simulink model "Powertrain_Model"  (R2021b)
settings: Solver=VariableStepAuto  StartTime=1  StopTime=sim_time  FixedStep=1  RelTol=1e-3
values from neighbouring files (symbols this model uses):
  a = (1-WD)*L    (= 1.352)    [Master_Script.m]
  airDen = 1.26    [Master_Script.m]
  b = WD*L    (= 1.248)    [Master_Script.m]
  Cd = 0.27    [Master_Script.m]
  contPowerRating = contPowerRating * numMotors    (= 400000)    [Master_Script.m]
  eff_batt = 0.9    [Master_Script.m]
  eff_trans = 0.95    [Master_Script.m]
  EM_Torque_Map = EM_Torque_Map * numMotors    [Master_Script.m]
  EM_Torque_Max = EM_Torque_Max * numMotors    [Master_Script.m]
  fArea = w103Dim*h101Dim    (= 2.727)    [Master_Script.m]
  followDriveCycle = 0    [Master_Script.m]
  fr = 0.009    [Master_Script.m]
  g = 9.81    [Master_Script.m]
  gearRatio = 8    [Master_Script.m]
  grade = 0    [Master_Script.m]    (also in isSetupSuitable.m = 0.12)
  h = 0.65    [Master_Script.m]
  isRWD = 0    [Master_Script.m]
  Ki = 0    [Master_Script.m]
  Kp = 1    [Master_Script.m]
  L = 2.6    [Master_Script.m]
  mu = 1    [Master_Script.m]
  mVehicle = originalmVehicle    (= 1372.4)    [Master_Script.m]
  netBattCap = capCell * numCellSeries * numParallelStrings    (= 52.224)    [Master_Script.m]
  R = 0.6681    [Master_Script.m]
undefined symbols (not defined in the file or in its folder): alpha, EM_Efficiency, EM_Omega_Map, EM_Omega_Max, t_cyc, v_cyc
libraries: slpidlib x1
settings Model: Creator=adity  LastModifiedBy=Shubham
settings SolverCC: AlgebraicLoopSolver=TrustRegion
settings DebuggingCC: SFMachineParentedDataDiag=warning
settings SFSimCC: CustomCodeUndefinedFunction=UseInterfaceOnly

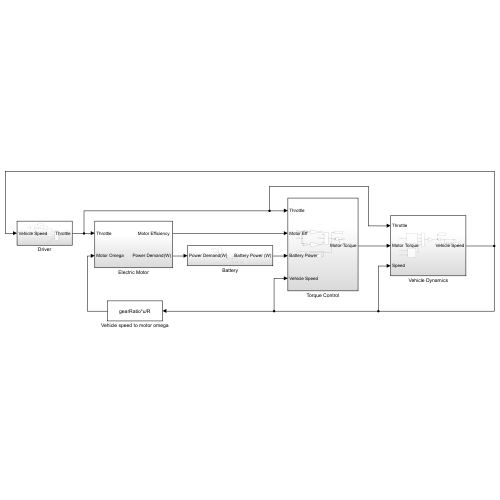
[thumbnail: Simulink's stored preview of the top-level diagram]
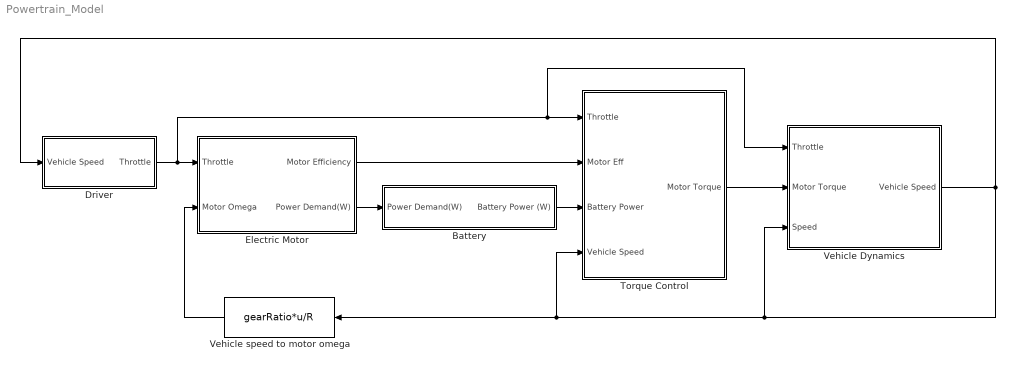
== system Powertrain_Model ==
  Battery : Subsystem
  Driver : Subsystem
  Electric Motor : Subsystem
  Torque Control : Subsystem
  Vehicle Dynamics : Subsystem
  Vehicle speed to motor omega : Fcn  Expr=gearRatio*u/R
  wires:
  Driver/1(Throttle) -> Vehicle Dynamics/1(Throttle), Torque Control/1(Throttle), Electric Motor/1("Throttle ")
  Vehicle speed to motor omega/1 -> Electric Motor/2(Motor Omega)
  Electric Motor/2(Power Demand(W)) -> Battery/1(Power Demand(W))
  Vehicle Dynamics/1(Vehicle Speed) -> Driver/1(Vehicle Speed), Vehicle Dynamics/3(Speed), Torque Control/4(Vehicle Speed), Vehicle speed to motor omega/1
  Battery/1(Battery Power (W)) -> Torque Control/3(Battery Power)
  Electric Motor/1("Motor Efficiency ") -> Torque Control/2(Motor Eff)
  Torque Control/1(Motor Torque) -> Vehicle Dynamics/2(Motor Torque)

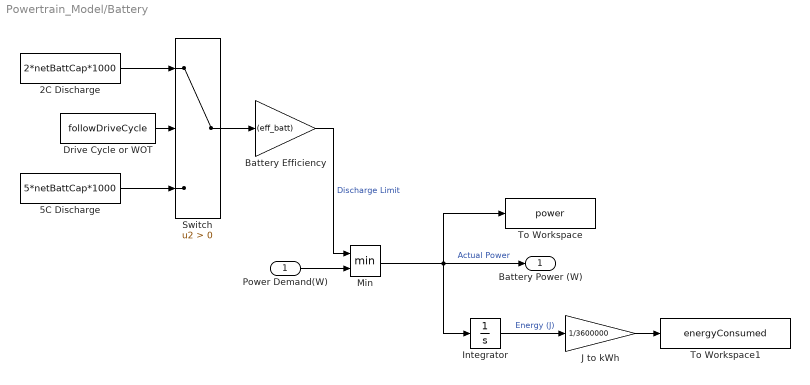
== system Powertrain_Model/Battery ==
  Power Demand(W) : Inport
  2C Discharge : Constant  Value=2*netBattCap*1000
  5C Discharge : Constant  Value=5*netBattCap*1000
  Battery Efficiency : Gain  Gain=(eff_batt)
  Drive Cycle or WOT : Constant  Value=followDriveCycle
  Integrator : Integrator
  J to kWh : Gain  Gain=1/3600000
  Min : MinMax  Inputs=2
  Switch : Switch  Criteria=u2 > Threshold
  To Workspace : ToWorkspace  VariableName=power  SaveFormat=Timeseries  SampleTime=-1
  To Workspace1 : ToWorkspace  VariableName=energyConsumed  SaveFormat=Timeseries  SampleTime=-1
  Battery Power (W) : Outport
  wires:
  Min/1 -> Battery Power (W)/1, To Workspace/1, Integrator/1  "Actual Power"
  Integrator/1 -> J to kWh/1  "Energy (J)"
  J to kWh/1 -> To Workspace1/1
  5C Discharge/1 -> Switch/3
  Battery Efficiency/1 -> Min/1  "Discharge Limit"
  Drive Cycle or WOT/1 -> Switch/2
  Switch/1 -> Battery Efficiency/1
  2C Discharge/1 -> Switch/1
  Power Demand(W)/1 -> Min/2

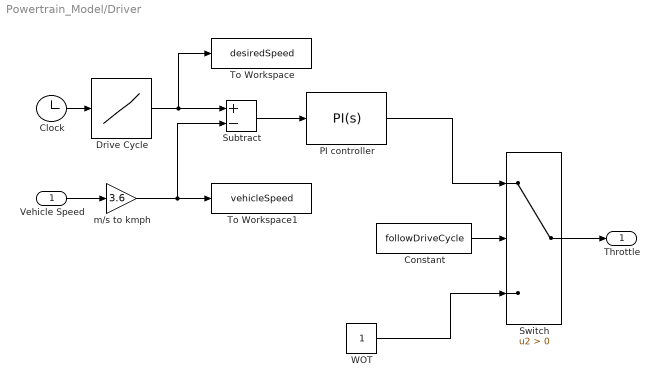
== system Powertrain_Model/Driver ==
  Vehicle Speed : Inport
  Clock : Clock
  Constant : Constant  Value=followDriveCycle
  Drive Cycle : Lookup_n-D  NumberOfTableDimensions=1  BreakpointsForDimension1=t_cyc  Table=v_cyc  InternalRulePriority=Speed  RndMeth=Simplest  InputSameDT=on
  "PI controller " : slpidlib/PID Controller  Controller=PI  Form=Parallel  TimeDomain=Continuous-time  UseExternalTs=off  SampleTime=-1  IntegratorMethod=Forward Euler  FilterMethod=Forward Euler  ControllerParametersSource=internal  P=Kp  I=Ki  D=0  UseFilter=on  N=100  TunerSelectOption=Transfer Function Based (PID Tuner App)  InitialConditionSource=internal  InitialConditionForIntegrator=0  InitialConditionForFilter=0  DifferentiatorICPrevScaledInput=0  ExternalReset=none  TrackingMode=off  Kt=1  LimitOutput=on  SatLimitsSource=internal  UpperSaturationLimit=1  LowerSaturationLimit=-1  LinearizeAsGain=on  AntiWindupMode=none  Kb=1  POutMin=[]  POutMax=[]  IOutMin=[]  IOutMax=[]  DOutMin=[]  DOutMax=[]  NOutMin=[]  NOutMax=[]  SumOutMin=[]  SumOutMax=[]  SaturationOutMin=[]  SaturationOutMax=[]  PParamMin=[]  PParamMax=[]  IParamMin=[]  IParamMax=[]  DParamMin=[]  DParamMax=[]  NParamMin=[]  NParamMax=[]  KbParamMin=[]  KbParamMax=[]  KtParamMin=[]  KtParamMax=[]  KbOutMin=[]  KbOutMax=[]  KtOutMin=[]  KtOutMax=[]  IntegratorOutMin=[]  IntegratorOutMax=[]  FilterOutMin=[]  FilterOutMax=[]  SumI1OutMin=[]  SumI1OutMax=[]  SumI2OutMin=[]  SumI2OutMax=[]  SumI3OutMin=[]  SumI3OutMax=[]  SumI4OutMin=[]  SumI4OutMax=[]  SumDOutMin=[]  SumDOutMax=[]  DifferentiatorOutMin=[]  DifferentiatorOutMax=[]  FilterDiffOutCoefMin=[]  FilterDiffOutCoefMax=[]  ReciprocalOutMin=[]  ReciprocalOutMax=[]  SumDenOutMin=[]  SumDenOutMax=[]  SumNumOutMin=[]  SumNumOutMax=[]  DivideOutMin=[]  DivideOutMax=[]  UdiffTsProdOutMin=[]  UdiffTsProdOutMax=[]  NTsProdOutMin=[]  NTsProdOutMax=[]  UintegralTsProdOutMin=[]  UintegralTsProdOutMax=[]  UngainTsProdOutMin=[]  UngainTsProdOutMax=[]  IntegratorContinuousStateAttributes=''  IntegratorStateMustResolveToSignalObject=off  IntegratorRTWStateStorageClass=Auto  FilterContinuousStateAttributes=''  FilterStateMustResolveToSignalObject=off  FilterRTWStateStorageClass=Auto  ParallelPVariant=InternalParameters  IdealPVariant=Disabled  IVariant=InternalParameters  DVariant=Disabled  IntegratorVariant=Continuous  SatVariant=Enabled  AWVariant=Passthrough  PCopyVariant=Disabled  TRVariant=Disabled  FdbkBlocksVariant=Forward  IdealPFdbkVariant=Disabled  SatFdbkVariant=Disabled  DerivativeFilterVariant=Disabled  NVariant=Disabled  NCopyVariant=Disabled_SignalSpec  FilterICVariant=Disabled  IntegratorICVariant=InternalICs  ExternalResetVariant=Disabled  TRSumVariant=Passthrough  SumFdbkVariant=Disabled  SumVariant=Sum_PI  TsampFilterVariant=InternalTs  TsampNgainVariant=Passthrough  TsampIntegralVariant=Passthrough  ExternalSaturationOutDataTypeStr=Inherit: Same as second input
  Subtract : Sum  Inputs=+-
  Switch : Switch  Criteria=u2 > Threshold
  To Workspace : ToWorkspace  VariableName=desiredSpeed  SaveFormat=Timeseries  SampleTime=-1
      settings: Save2DSignal=2-D array (concatenate along first dimension)
  To Workspace1 : ToWorkspace  VariableName=vehicleSpeed  SaveFormat=Timeseries  SampleTime=-1
  WOT : Constant
  m/s to kmph : Gain  Gain=3.6
  Throttle : Outport
  wires:
  Drive Cycle/1 -> Subtract/1, To Workspace/1
  Subtract/1 -> "PI controller "/1
  Clock/1 -> Drive Cycle/1
  Switch/1 -> Throttle/1
  "PI controller "/1 -> Switch/1
  Constant/1 -> Switch/2
  WOT/1 -> Switch/3
  Vehicle Speed/1 -> m/s to kmph/1
  m/s to kmph/1 -> To Workspace1/1, Subtract/2

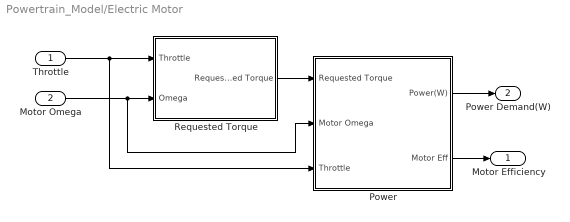
== system Powertrain_Model/Electric Motor ==
  "Throttle " : Inport
  Motor Omega : Inport  Port=2
  Power : Subsystem
  Requested Torque : Subsystem
  "Motor Efficiency " : Outport
  Power Demand(W) : Outport  Port=2
  wires:
  Requested Torque/1(Requested Torque) -> Power/1(Requested Torque)
  "Throttle "/1 -> Requested Torque/1(Throttle), Power/3("Throttle ")
  Power/1("Power(W) ") -> Power Demand(W)/1
  Motor Omega/1 -> Requested Torque/2(Omega), Power/2(Motor Omega)
  Power/2(Motor Eff) -> "Motor Efficiency "/1

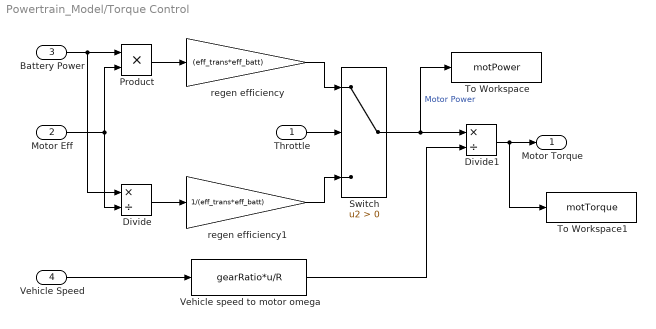
== system Powertrain_Model/Torque Control ==
  Throttle : Inport
  Motor Eff : Inport  Port=2
  Battery Power : Inport  Port=3
  Vehicle Speed : Inport  Port=4
  Divide : Product  Inputs=*/
  Divide1 : Product  Inputs=*/
  Product : Product
  Switch : Switch  Criteria=u2 > Threshold
  To Workspace : ToWorkspace  VariableName=motPower  SaveFormat=Timeseries  SampleTime=-1
  To Workspace1 : ToWorkspace  VariableName=motTorque  SaveFormat=Timeseries  SampleTime=-1
  Vehicle speed to motor omega : Fcn  Expr=gearRatio*u/R
  regen efficiency : Gain  Gain=(eff_trans*eff_batt)
  regen efficiency1 : Gain  Gain=1/(eff_trans*eff_batt)
  Motor Torque : Outport
  wires:
  Throttle/1 -> Switch/2
  Battery Power/1 -> Product/1, Divide/1
  Motor Eff/1 -> Divide/2, Product/2
  Product/1 -> regen efficiency/1
  Divide/1 -> regen efficiency1/1
  regen efficiency/1 -> Switch/1
  regen efficiency1/1 -> Switch/3
  Switch/1 -> To Workspace/1, Divide1/1  "Motor Power"
  Vehicle Speed/1 -> Vehicle speed to motor omega/1
  Divide1/1 -> To Workspace1/1, Motor Torque/1
  Vehicle speed to motor omega/1 -> Divide1/2

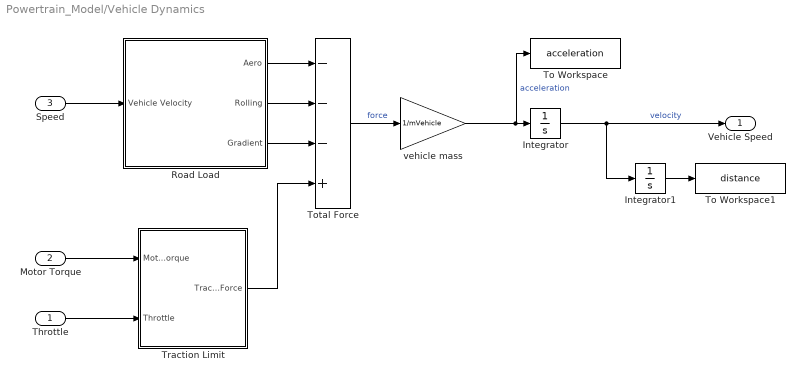
== system Powertrain_Model/Vehicle Dynamics ==
  Throttle : Inport
  Motor Torque : Inport  Port=2
  Speed : Inport  Port=3
  Integrator : Integrator
  Integrator1 : Integrator
  Road Load : Subsystem
  To Workspace : ToWorkspace  VariableName=acceleration  SaveFormat=Timeseries  SampleTime=-1
  To Workspace1 : ToWorkspace  VariableName=distance  SaveFormat=Timeseries  SampleTime=-1
  Total Force : Sum  Inputs=---+
  Traction Limit : Subsystem
  vehicle mass : Gain  Gain=1/mVehicle
  Vehicle Speed : Outport
  wires:
  Road Load/3(Gradient) -> Total Force/3
  Road Load/2(Rolling) -> Total Force/2
  Road Load/1("Aero ") -> Total Force/1
  Speed/1 -> Road Load/1(Vehicle Velocity)
  Motor Torque/1 -> Traction Limit/1(Motor Torque)
  Throttle/1 -> Traction Limit/2(Throttle)
  Traction Limit/1(Traction Force) -> Total Force/4
  Total Force/1 -> vehicle mass/1  "force"
  vehicle mass/1 -> To Workspace/1, Integrator/1  "acceleration"
  Integrator/1 -> Vehicle Speed/1, Integrator1/1  "velocity"
  Integrator1/1 -> To Workspace1/1

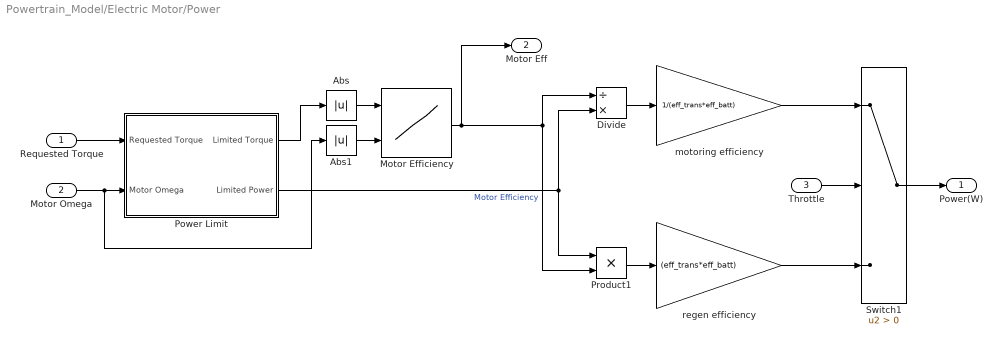
== system Powertrain_Model/Electric Motor/Power ==
  Requested Torque : Inport
  Motor Omega : Inport  Port=2
  "Throttle " : Inport  Port=3
  Abs : Abs
  Abs1 : Abs
  Divide : Product  Inputs=/*
  Motor Efficiency : Lookup_n-D  BreakpointsForDimension1=EM_Torque_Map  BreakpointsForDimension2=EM_Omega_Map  Table=EM_Efficiency  InternalRulePriority=Speed  RndMeth=Simplest  InputSameDT=on
      settings: InputPortMap=u0,u1
  Power Limit : Subsystem
  Product1 : Product
  Switch1 : Switch  Criteria=u2 > Threshold
  motoring efficiency : Gain  Gain=1/(eff_trans*eff_batt)
  regen efficiency : Gain  Gain=(eff_trans*eff_batt)
  "Power(W) " : Outport
  Motor Eff : Outport  Port=2
  wires:
  regen efficiency/1 -> Switch1/3
  motoring efficiency/1 -> Switch1/1
  Product1/1 -> regen efficiency/1
  Divide/1 -> motoring efficiency/1
  Switch1/1 -> "Power(W) "/1
  "Throttle "/1 -> Switch1/2
  Motor Efficiency/1 -> Divide/1, Product1/2, Motor Eff/1  "Motor Efficiency"
  Abs/1 -> Motor Efficiency/1
  Abs1/1 -> Motor Efficiency/2
  Requested Torque/1 -> Power Limit/1(Requested Torque)
  Motor Omega/1 -> Power Limit/2(Motor Omega), Abs1/1
  Power Limit/1(Limited Torque) -> Abs/1
  Power Limit/2(Limited Power) -> Product1/1, Divide/2

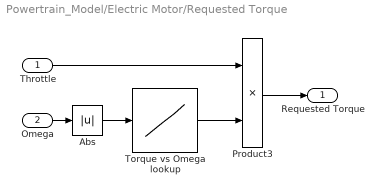
== system Powertrain_Model/Electric Motor/Requested Torque ==
  Throttle : Inport
  Omega : Inport  Port=2
  Abs : Abs
  Product3 : Product  RndMeth=Zero
  Torque vs Omega lookup : Lookup_n-D  NumberOfTableDimensions=1  BreakpointsForDimension1=EM_Omega_Max  BreakpointsForDimension2=alpha  Table=EM_Torque_Max  InternalRulePriority=Speed  RndMeth=Simplest  InputSameDT=on
  Requested Torque : Outport
  wires:
  Product3/1 -> Requested Torque/1
  Throttle/1 -> Product3/1
  Torque vs Omega lookup/1 -> Product3/2
  Omega/1 -> Abs/1
  Abs/1 -> Torque vs Omega lookup/1

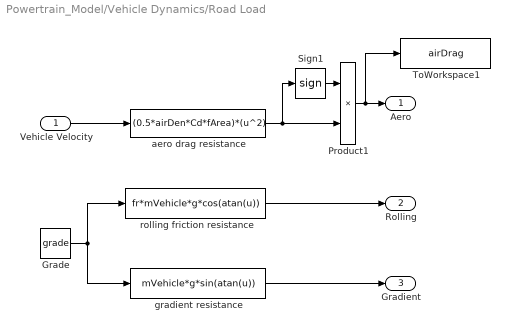
== system Powertrain_Model/Vehicle Dynamics/Road Load ==
  Vehicle Velocity : Inport
  Grade : Constant  Value=grade
  Product1 : Product
  Sign1 : Signum
  ToWorkspace1 : ToWorkspace  VariableName=airDrag  SaveFormat=Timeseries  SampleTime=-1
      settings: Save2DSignal=2-D array (concatenate along first dimension)
  aero drag resistance : Fcn  Expr=(0.5*airDen*Cd*fArea)*(u^2)
  gradient resistance : Fcn  Expr=mVehicle*g*sin(atan(u))
  rolling friction resistance : Fcn  Expr=fr*mVehicle*g*cos(atan(u))
  "Aero " : Outport
  Rolling : Outport  Port=2
  Gradient : Outport  Port=3
  wires:
  Grade/1 -> gradient resistance/1, rolling friction resistance/1
  rolling friction resistance/1 -> Rolling/1
  gradient resistance/1 -> Gradient/1
  Sign1/1 -> Product1/1
  Vehicle Velocity/1 -> aero drag resistance/1
  Product1/1 -> ToWorkspace1/1, "Aero "/1
  aero drag resistance/1 -> Product1/2, Sign1/1

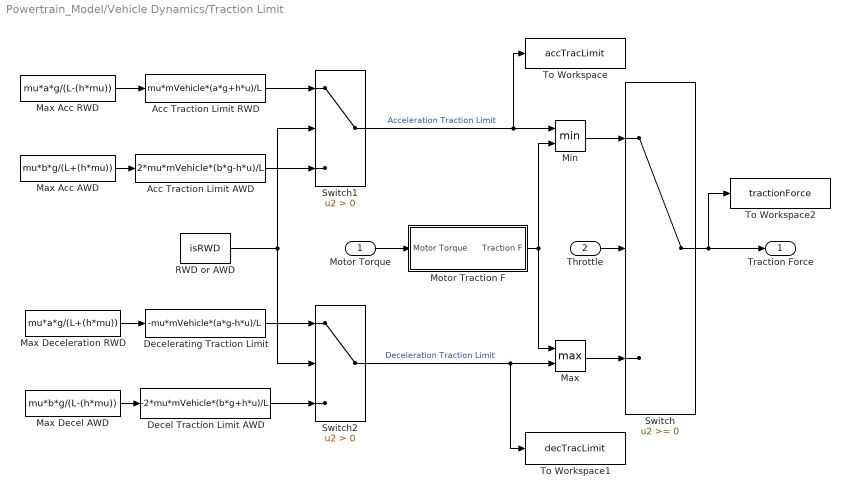
== system Powertrain_Model/Vehicle Dynamics/Traction Limit ==
  Motor Torque : Inport
  Throttle : Inport  Port=2
  Acc Traction Limit AWD : Fcn  Expr=2*mu*mVehicle*(b*g-h*u)/L
  Acc Traction Limit RWD : Fcn  Expr=mu*mVehicle*(a*g+h*u)/L
  Decel Traction Limit AWD : Fcn  Expr=-2*mu*mVehicle*(b*g+h*u)/L
  Decelerating Traction Limit : Fcn  Expr=-mu*mVehicle*(a*g-h*u)/L
  Max : MinMax  Function=max  Inputs=2
  Max Acc AWD : Constant  Value=mu*b*g/(L+(h*mu))
  Max Acc RWD : Constant  Value=mu*a*g/(L-(h*mu))
  Max Decel AWD : Constant  Value=mu*b*g/(L-(h*mu))
  Max Deceleration RWD : Constant  Value=mu*a*g/(L+(h*mu))
  Min : MinMax  Inputs=2
  Motor Traction F : Subsystem
  RWD or AWD : Constant  Value=isRWD
  Switch : Switch
  Switch1 : Switch  Criteria=u2 > Threshold
  Switch2 : Switch  Criteria=u2 > Threshold
  To Workspace : ToWorkspace  VariableName=accTracLimit  SaveFormat=Timeseries  SampleTime=-1
  To Workspace1 : ToWorkspace  VariableName=decTracLimit  SaveFormat=Timeseries  SampleTime=-1
  To Workspace2 : ToWorkspace  VariableName=tractionForce  SaveFormat=Timeseries  SampleTime=-1
  Traction Force : Outport
  wires:
  Switch1/1 -> To Workspace/1, Min/1  "Acceleration Traction Limit"
  Switch2/1 -> To Workspace1/1, Max/2  "Deceleration Traction Limit"
  Max Acc RWD/1 -> Acc Traction Limit RWD/1
  Acc Traction Limit RWD/1 -> Switch1/1
  Decelerating Traction Limit/1 -> Switch2/1
  Max Decel AWD/1 -> Decel Traction Limit AWD/1
  Decel Traction Limit AWD/1 -> Switch2/3
  RWD or AWD/1 -> Switch1/2, Switch2/2
  Max Deceleration RWD/1 -> Decelerating Traction Limit/1
  Max Acc AWD/1 -> Acc Traction Limit AWD/1
  Acc Traction Limit AWD/1 -> Switch1/3
  Min/1 -> Switch/1
  Motor Traction F/1(Traction F) -> Min/2, Max/1
  Max/1 -> Switch/3
  Throttle/1 -> Switch/2
  Switch/1 -> Traction Force/1, To Workspace2/1
  Motor Torque/1 -> Motor Traction F/1(Motor Torque)

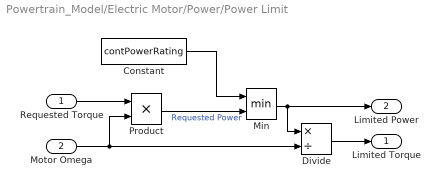
== system Powertrain_Model/Electric Motor/Power/Power Limit ==
  Requested Torque : Inport
  Motor Omega : Inport  Port=2
  Constant : Constant  Value=contPowerRating
  Divide : Product  Inputs=*/
  Min : MinMax  Inputs=2
  Product : Product
  Limited Torque : Outport
  Limited Power : Outport  Port=2
  wires:
  Product/1 -> Min/2  "Requested Power"
  Motor Omega/1 -> Divide/2, Product/2
  Constant/1 -> Min/1
  Min/1 -> Divide/1, Limited Power/1
  Divide/1 -> Limited Torque/1
  Requested Torque/1 -> Product/1

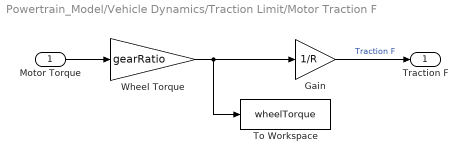
== system Powertrain_Model/Vehicle Dynamics/Traction Limit/Motor Traction F ==
  Motor Torque : Inport
  Gain : Gain  Gain=1/R
  To Workspace : ToWorkspace  VariableName=wheelTorque  SaveFormat=Timeseries  SampleTime=-1
  Wheel Torque : Gain  Gain=gearRatio
  Traction F : Outport
  wires:
  Wheel Torque/1 -> To Workspace/1, Gain/1
  Motor Torque/1 -> Wheel Torque/1
  Gain/1 -> Traction F/1  "Traction F"
